simulink model "Plant"  (R2018b)
settings: configuration reference "plant_config" (kept outside this file)
values from neighbouring files (symbols this model uses):
  PLANT_EXPORT = Simulink.Parameter(PLANT_EXPORT_VALUE)    [multicopter_model_init.m]    (also in plant_model_init.m)
undefined symbols (not defined in the file or in its folder): acc_x, acc_x_O, acc_y, acc_y_O, acc_z, acc_z_O, alt, alt_ref, day, DiscIntNeverNeededParam, fixType, flags, gSpeed, gyr_x, gyr_y, gyr_z, h_R, hAcc, headAcc, headMot, height, hMSL, hour, iTOW, lat, lat_ref, lon, lon_ref, M_BO, M_OB, mag_x, mag_y, mag_z, month, nano, Newton, numSV, pDOP, phi, PLANT_CONST, plant_model, pressure, prop_vel, psi, quat, Raphson, reserved1, reserved2, rot_x_B, rot_y_B, rot_z_B, sAcc, sec, Sensor_Model, tAcc, temperature, temprature, theta, timestamp, vAcc ... (+10)
libraries: simulink x6, dspsrcs4 x6, AP_Math x3, Quaternion x3, Rotation x2, aerolibatmos2 x1
(part 1 of 2)
settings Model: Creator=zouji  LastModifiedBy=zouji
settings ConfigSetRef: SourceLocation=Base Workspace

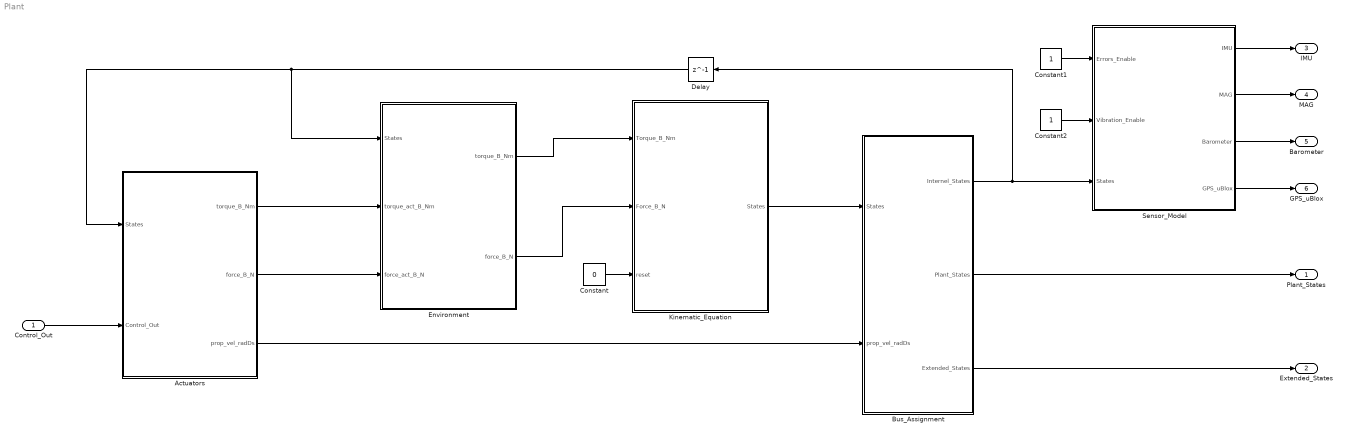
== system Plant ==
  Control_Out : Inport  OutDataTypeStr=Bus: Control_Out_Bus
  Actuators : Subsystem  TreatAsAtomicUnit=on
  Bus_Assignment : Subsystem  TreatAsAtomicUnit=on  mask{lon_0=0.65673, lat_0=-2.1361, hgt_0=4.5}
      mask prompts: lon_0 "init lontitude (rad)"; lat_0 "init latitude (rad)"; hgt_0 "init height (m)"
  Constant : Constant  Value=0  OutDataTypeStr=Inherit: Inherit via back propagation
  Constant1 : Constant  OutDataTypeStr=Inherit: Inherit via back propagation
  Constant2 : Constant  OutDataTypeStr=Inherit: Inherit via back propagation
  Delay : Delay  DelayLength=1
  Environment : Subsystem  TreatAsAtomicUnit=on
  Kinematic_Equation : Subsystem  TreatAsAtomicUnit=on
  Sensor_Model : Subsystem  TreatAsAtomicUnit=on
  Plant_States : Outport  OutDataTypeStr=Bus: Plant_States_Bus
  Extended_States : Outport  Port=2  OutDataTypeStr=Bus: Extended_States_Bus
  IMU : Outport  Port=3  OutDataTypeStr=Bus: IMU_Bus
  MAG : Outport  Port=4  OutDataTypeStr=Bus: MAG_Bus
  Barometer : Outport  Port=5  OutDataTypeStr=Bus: Barometer_Bus
  GPS_uBlox : Outport  Port=6  OutDataTypeStr=Bus: GPS_uBlox_Bus
  wires:
  Kinematic_Equation/1(States) -> Bus_Assignment/1(States)
  Control_Out/1 -> Actuators/2(Control_Out)
  Bus_Assignment/2(Plant_States) -> Plant_States/1
  Constant1/1 -> Sensor_Model/1(Errors_Enable)
  Sensor_Model/1(IMU) -> IMU/1
  Sensor_Model/2(MAG) -> MAG/1
  Sensor_Model/3(Barometer) -> Barometer/1
  Sensor_Model/4(GPS_uBlox) -> GPS_uBlox/1
  Actuators/3(prop_vel_radDs) -> Bus_Assignment/2(prop_vel_radDs)
  Delay/1 -> Environment/1(States), Actuators/1(States)
  Constant2/1 -> Sensor_Model/2(Vibration_Enable)
  Actuators/1(torque_B_Nm) -> Environment/2(torque_act_B_Nm)
  Actuators/2(force_B_N) -> Environment/3(force_act_B_N)
  Environment/1(torque_B_Nm) -> Kinematic_Equation/1(Torque_B_Nm)
  Environment/2(force_B_N) -> Kinematic_Equation/2(Force_B_N)
  Constant/1 -> Kinematic_Equation/3(reset)
  Bus_Assignment/3(Extended_States) -> Extended_States/1
  Bus_Assignment/1(Internel_States) -> Sensor_Model/3(States), Delay/1

== system Plant/Actuators ==
  States : Inport
  Control_Out : Inport  Port=2
  Aerodynamic : Subsystem
  Bus Selector : BusSelector  OutputSignals=Plant_States.rot_x_B,Plant_States.rot_y_B,Plant_States.rot_z_B
  Motors : Subsystem
  Mux : Mux  Inputs=3
  Sum : Sum  Inputs=|++
  torque_B_Nm : Outport
  force_B_N : Outport  Port=2
  prop_vel_radDs : Outport  Port=3
  wires:
  Control_Out/1 -> Motors/1(Control_Out)
  States/1 -> Aerodynamic/1(States), Bus Selector/1
  Motors/1(torque_B_Nm) -> torque_B_Nm/1
  Motors/2(force_B_N) -> Sum/1
  Motors/3(prop_vel_radDs) -> prop_vel_radDs/1
  Bus Selector/1 -> Mux/1  "<rot_x_B>"
  Bus Selector/2 -> Mux/2  "<rot_y_B>"
  Bus Selector/3 -> Mux/3  "<rot_z_B>"
  Mux/1 -> Motors/2(omega_B_radDs)
  Sum/1 -> force_B_N/1
  Aerodynamic/1(aero_force_B_N) -> Sum/2

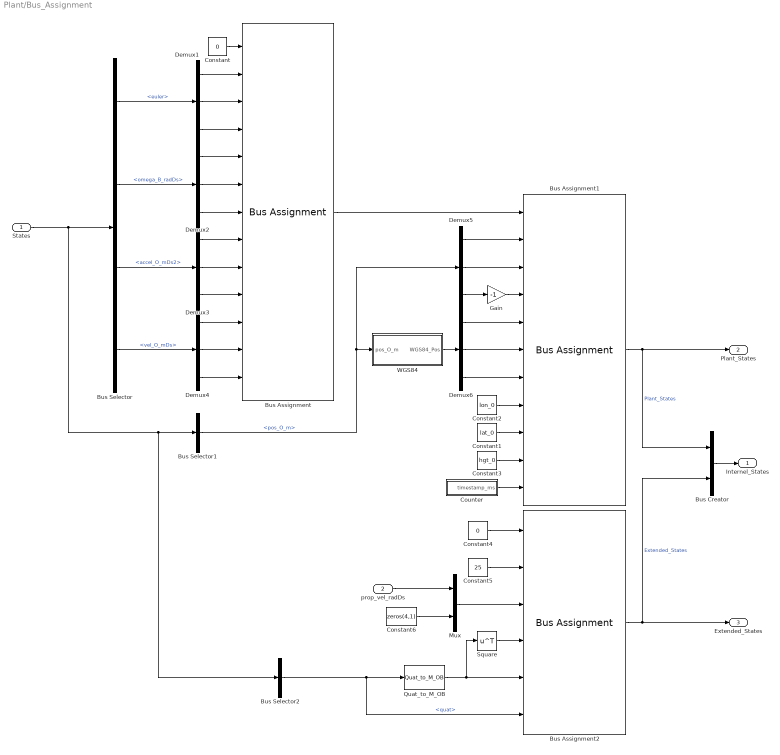
== system Plant/Bus_Assignment ==
  States : Inport
  prop_vel_radDs : Inport  Port=2
  Bus Assignment : BusAssignment  AssignedSignals=phi,theta,psi,rot_x_B,rot_y_B,rot_z_B,acc_x_O,acc_y_O,acc_z_O,vel_x_O,vel_y_O,vel_z_O
  Bus Assignment1 : BusAssignment  AssignedSignals=x_R,y_R,h_R,lat,lon,alt,lon_ref,lat_ref,alt_ref,timestamp
  Bus Assignment2 : BusAssignment  AssignedSignals=temprature,prop_vel,M_BO,M_OB,quat
  Bus Creator : BusCreator  Inputs=2
  Bus Selector : BusSelector  OutputSignals=euler,omega_B_radDs,accel_O_mDs2,vel_O_mDs
  Bus Selector1 : BusSelector  OutputSignals=pos_O_m
  Bus Selector2 : BusSelector  OutputSignals=quat
  Constant : Constant  Value=0  OutDataTypeStr=Bus: Plant_States_Bus
  Constant1 : Constant  Value=lat_0
  Constant2 : Constant  Value=lon_0
  Constant3 : Constant  Value=hgt_0
  Constant4 : Constant  Value=0  OutDataTypeStr=Bus: Extended_States_Bus
  Constant5 : Constant  Value=25  OutDataTypeStr=Inherit: Inherit via back propagation
  Constant6 : Constant  Value=zeros(4,1)  OutDataTypeStr=single
  Counter : Subsystem
  Demux{1..6} (6 alike) : Demux  Outputs=3
  Gain : Gain  Gain=-1  OutDataTypeStr=Inherit: Same as input
  Mux : Mux  Inputs=2
  Quat_to_M_OB : Rotation/Quat_to_M_OB  SystemSampleTime=-1
  Square : Math  Operator=transpose  SaturateOnIntegerOverflow=on
  WGS84 : Subsystem
  Internel_States : Outport
  Plant_States : Outport  Port=2
  Extended_States : Outport  Port=3
  wires:
  Constant/1 -> Bus Assignment/1
  States/1 -> Bus Selector2/1, Bus Selector1/1, Bus Selector/1
  Bus Selector/1 -> Demux1/1  "<euler>"
  Bus Selector/2 -> Demux2/1  "<omega_B_radDs>"
  Bus Selector/3 -> Demux3/1  "<accel_O_mDs2>"
  Bus Selector/4 -> Demux4/1  "<vel_O_mDs>"
  Bus Assignment/1 -> Bus Assignment1/1
  Bus Selector1/1 -> Demux5/1, WGS84/1(pos_O_m)  "<pos_O_m>"
  Bus Assignment1/1 -> Plant_States/1, Bus Creator/1  "Plant_States"
  Quat_to_M_OB/1 -> Bus Assignment2/5, Square/1
  Demux1/2 -> Bus Assignment/3
  prop_vel_radDs/1 -> Mux/1
  Demux5/3 -> Gain/1
  WGS84/1(WGS84_Pos) -> Demux6/1
  Demux1/1 -> Bus Assignment/2
  Demux1/3 -> Bus Assignment/4
  Demux2/1 -> Bus Assignment/5
  Demux2/2 -> Bus Assignment/6
  Demux2/3 -> Bus Assignment/7
  Demux3/1 -> Bus Assignment/8
  Demux3/2 -> Bus Assignment/9
  Demux3/3 -> Bus Assignment/10
  Demux4/1 -> Bus Assignment/11
  Demux4/2 -> Bus Assignment/12
  Demux4/3 -> Bus Assignment/13
  Demux5/2 -> Bus Assignment1/3
  Gain/1 -> Bus Assignment1/4
  Demux5/1 -> Bus Assignment1/2
  Demux6/1 -> Bus Assignment1/5
  Demux6/2 -> Bus Assignment1/6
  Demux6/3 -> Bus Assignment1/7
  Constant2/1 -> Bus Assignment1/8
  Constant1/1 -> Bus Assignment1/9
  Constant3/1 -> Bus Assignment1/10
  Constant4/1 -> Bus Assignment2/1
  Constant5/1 -> Bus Assignment2/2
  Mux/1 -> Bus Assignment2/3
  Constant6/1 -> Mux/2
  Square/1 -> Bus Assignment2/4
  Bus Selector2/1 -> Quat_to_M_OB/1, Bus Assignment2/6  "<quat>"
  Bus Assignment2/1 -> Bus Creator/2, Extended_States/1  "Extended_States"
  Bus Creator/1 -> Internel_States/1
  Counter/1(timestamp_ms) -> Bus Assignment1/11

== system Plant/Environment ==
  States : Inport
  torque_act_B_Nm : Inport  Port=2
  force_act_B_N : Inport  Port=3
  Add : Sum  Inputs=+++
  Add1 : Sum
  Gravity : Subsystem
  Ground_Model : Subsystem
  torque_B_Nm : Outport
  force_B_N : Outport  Port=2
  wires:
  States/1 -> Ground_Model/1(States), Gravity/1(States)
  Gravity/1(g_B_N) -> Add/2
  force_act_B_N/1 -> Add/3
  Ground_Model/2(force_gnd_B_N) -> Add/1
  Add/1 -> force_B_N/1
  Ground_Model/1(torque_gnd_B_Nm) -> Add1/2
  torque_act_B_Nm/1 -> Add1/1
  Add1/1 -> torque_B_Nm/1

== system Plant/Kinematic_Equation ==
  Torque_B_Nm : Inport
  Force_B_N : Inport  Port=2
  reset : Inport  Port=3
  Attitude_Dynamic : Subsystem  mask{Ixx=plant_model.Jxx, Iyy=plant_model.Jyy, Izz=plant_model.Jzz}
  Bus Creator : BusCreator  Inputs=7
  Position_Dynamic : Subsystem  mask{mass=plant_model.mass}
  States : Outport
  wires:
  Attitude_Dynamic/2(omega_B_radDs) -> Bus Creator/2, Position_Dynamic/2(omega_B_radDs)  "omega_B_radDs"
  Attitude_Dynamic/3(quat) -> Bus Creator/3, Position_Dynamic/3(quat)  "quat"
  reset/1 -> Attitude_Dynamic/2(reset), Position_Dynamic/4(vel_reset)
  Bus Creator/1 -> States/1  "states"
  Attitude_Dynamic/1(dot_omega_B_radDs2) -> Bus Creator/1  "dot_omega_B_radDs2"
  Attitude_Dynamic/4(euler) -> Bus Creator/4  "euler"
  Position_Dynamic/1(accel_O_mDs2) -> Bus Creator/5  "accel_O_mDs2"
  Position_Dynamic/2(vel_O_mDs) -> Bus Creator/6  "vel_O_mDs"
  Position_Dynamic/3(pos_NED_O_m) -> Bus Creator/7  "pos_O_m"
  Force_B_N/1 -> Position_Dynamic/1(force_B_N)
  Torque_B_Nm/1 -> Attitude_Dynamic/1(torque_B_Nm)

== system Plant/Sensor_Model ==
  Errors_Enable : Inport  OutDataTypeStr=uint8
  Vibration_Enable : Inport  Port=2  OutDataTypeStr=uint8
  States : Inport  Port=3
  Counter : Subsystem
  Sensor_Barometer : Subsystem  TreatAsAtomicUnit=on
  Sensor_GPS : Subsystem  TreatAsAtomicUnit=on
  Sensor_IMU : Subsystem  TreatAsAtomicUnit=on
  Sensor_MAG : Subsystem  TreatAsAtomicUnit=on
  IMU : Outport
  MAG : Outport  Port=2
  Barometer : Outport  Port=3
  GPS_uBlox : Outport  Port=4
  wires:
  Counter/1(timestamp_ms) -> Sensor_Barometer/3(timestamp_ms), Sensor_MAG/3(timestamp_ms), Sensor_IMU/4(timestamp_ms), Sensor_GPS/3(timestamp_ms)
  States/1 -> Sensor_GPS/1(States), Sensor_Barometer/1(States), Sensor_MAG/1(States), Sensor_IMU/1(States)
  Sensor_Barometer/1(Barometer) -> Barometer/1
  Sensor_MAG/1(Mag) -> MAG/1
  Sensor_IMU/1(IMU) -> IMU/1
  Vibration_Enable/1 -> Sensor_IMU/3(Vibration_Enable)
  Errors_Enable/1 -> Sensor_IMU/2(Errors_Enable), Sensor_GPS/2(Errors_Enable), Sensor_Barometer/2(Errors_Enable), Sensor_MAG/2(Errors_Enable)
  Sensor_GPS/1(GPS_uBlox) -> GPS_uBlox/1

== system Plant/Actuators/Aerodynamic ==
  States : Inport
  Air_Drag : Subsystem
  aero_force_B_N : Outport
  wires:
  States/1 -> Air_Drag/1(Plant_States)
  Air_Drag/1(air_drag_B) -> aero_force_B_N/1

== system Plant/Actuators/Motors ==
  Control_Out : Inport
  omega_B_radDs : Inport  Port=2
  ESCs : Subsystem  mask{T=plant_model.motorT, k=plant_model.motorCr, p=plant_model.motorWb}
  Force : Subsystem
  Torque : Subsystem
  torque_B_Nm : Outport
  force_B_N : Outport  Port=2
  prop_vel_radDs : Outport  Port=3
  wires:
  ESCs/1(rotor_speed_radDs) -> prop_vel_radDs/1, Force/1(rotor_speed_radDs), Torque/1(rotor_speed_radDs)  "prop_vel"
  omega_B_radDs/1 -> Torque/2(omega_B_radDs)
  Control_Out/1 -> ESCs/1(Control_Out)
  Torque/1(torque_B_Nm) -> torque_B_Nm/1
  Force/1(force_B_N) -> force_B_N/1

== system Plant/Bus_Assignment/Counter ==
  note: Careful: If change memory to delay,
      | that model will crash
  Data Type Conversion2 : DataTypeConversion  OutDataTypeStr=uint32
  Memory1 : Memory
  Sum : Sum  Inputs=|++
  dt : Constant  Value=PLANT_EXPORT.period  OutDataTypeStr=uint32
  timestamp_ms : Outport
  wires:
  dt/1 -> Sum/1
  Sum/1 -> Memory1/1
  Memory1/1 -> Sum/2, Data Type Conversion2/1
  Data Type Conversion2/1 -> timestamp_ms/1

== system Plant/Bus_Assignment/WGS84 ==
  pos_O_m : Inport
  Add : Sum
  Data Type Conversion : DataTypeConversion  OutDataTypeStr=double
  Delay : Delay  DelayLength=1
  Delay1 : Delay  DelayLength=1  InitialCondition=[lon_0;lat_0;hgt_0]
  Demux : Demux  Outputs=3
  Divide : Product  Inputs=/*
  Mux : Mux  Inputs=3
  Subtract : Sum  Inputs=+-
  Terminator : Terminator
  WGS84_Derivatives : Subsystem
  Zero_Value_Exclusion : Subsystem  mask{thr=1e-6}
      mask prompts: thr "Threshold"
      mask Display: disp('Exclude Zero');
  WGS84_Pos : Outport
  wires:
  pos_O_m/1 -> Data Type Conversion/1
  Delay/1 -> Subtract/2
  WGS84_Derivatives/1(dx_dlat) -> Mux/1
  Mux/1 -> Zero_Value_Exclusion/1(u)
  Zero_Value_Exclusion/1(y) -> Divide/1
  WGS84_Derivatives/3(dz_dh) -> Mux/3
  WGS84_Derivatives/2(dy_dlon) -> Mux/2
  Subtract/1 -> Divide/2
  Divide/1 -> Add/1
  Delay1/1 -> Demux/1, Add/2
  Add/1 -> Delay1/1, WGS84_Pos/1
  Demux/1 -> WGS84_Derivatives/1(lat_0)
  Demux/3 -> WGS84_Derivatives/2(h_0)
  Demux/2 -> Terminator/1
  Data Type Conversion/1 -> Delay/1, Subtract/1

== system Plant/Environment/Gravity ==
  States : Inport
  Bus Selector4 : BusSelector  OutputSignals=Extended_States.M_BO
  Multiply3 : Product  Multiplication=Matrix(*)
  mg : Constant  Value=[0;0;9.81*plant_model.mass]  OutDataTypeStr=single
  g_B_N : Outport
  wires:
  States/1 -> Bus Selector4/1
  Bus Selector4/1 -> Multiply3/1  "<M_BO>"
  Multiply3/1 -> g_B_N/1
  mg/1 -> Multiply3/2

== system Plant/Environment/Ground_Model ==
  States : Inport
  Bus Selector : BusSelector  OutputSignals=Plant_States.h_R
  Compare To Zero : simulink/Logic and Bit Operations/Compare To Zero  relop=<=  OutDataTypeStr=boolean
  Constant : Constant  Value=[0;0;0]  VectorParams1D=off  OutDataTypeStr=single
  Constant1 : Constant  Value=[0;0;0]  VectorParams1D=off  OutDataTypeStr=single
  Ground_Force : Subsystem
  Ground_Torque : Subsystem
  Switch1 : Switch  Criteria=u2 > Threshold
  Switch2 : Switch  Criteria=u2 > Threshold
  torque_gnd_B_Nm : Outport
  force_gnd_B_N : Outport  Port=2
  wires:
  Compare To Zero/1 -> Switch1/2, Switch2/2
  Constant/1 -> Switch2/3
  Switch2/1 -> force_gnd_B_N/1
  States/1 -> Ground_Force/1(States), Bus Selector/1, Ground_Torque/1(States)
  Bus Selector/1 -> Compare To Zero/1  "<h_R>"
  Ground_Force/1(force_gnd_B_N) -> Switch2/1
  Ground_Torque/1(torque_gnd_B_Nm) -> Switch1/1
  Constant1/1 -> Switch1/3
  Switch1/1 -> torque_gnd_B_Nm/1

== system Plant/Kinematic_Equation/Attitude_Dynamic ==
  torque_B_Nm : Inport
  reset : Inport  Port=2
  Constant1 : Constant  Value=[1;0;0;0]  OutDataTypeStr=single
  Discrete-Time Integrator : DiscreteIntegrator  ExternalReset=level  InitialCondition=[0;0;0]  SampleTime=-1  ICPrevOutput=DiscIntNeverNeededParam  ICPrevScaledInput=DiscIntNeverNeededParam
  Divide : Product  Inputs=/*  Multiplication=Matrix(*)  OutDataTypeStr=Inherit: Same as first input
  Inertia_Matrix : Constant  Value=[Ixx 0 0;0 Iyy 0;0 0 Izz]  OutDataTypeStr=single
  Multiply : Product  Multiplication=Matrix(*)  OutDataTypeStr=Inherit: Same as first input
  Quaternuin_Update : Subsystem
  Sum : Sum  Inputs=|+-  OutDataTypeStr=Inherit: Same as first input
  cross_product : AP_Math/cross_product  SystemSampleTime=-1
  quat to euler : Quaternion/quat to euler  SystemSampleTime=-1
  dot_omega_B_radDs2 : Outport
  omega_B_radDs : Outport  Port=2
  quat : Outport  Port=3
  euler : Outport  Port=4
  wires:
  Constant1/1 -> Quaternuin_Update/3(init_quat)
  quat to euler/1 -> euler/1
  Quaternuin_Update/1(quat) -> quat to euler/1, quat/1
  reset/1 -> Quaternuin_Update/2(reset), Discrete-Time Integrator/2
  Divide/1 -> dot_omega_B_radDs2/1, Discrete-Time Integrator/1  "dot_omega_B_radDs2"
  Sum/1 -> Divide/2
  cross_product/1 -> Sum/2
  torque_B_Nm/1 -> Sum/1
  Multiply/1 -> cross_product/2
  Inertia_Matrix/1 -> Multiply/1, Divide/1
  Discrete-Time Integrator/1 -> omega_B_radDs/1, Multiply/2, cross_product/1, Quaternuin_Update/1(omega_B_radDs)  "omega_B_radDs"

== system Plant/Kinematic_Equation/Position_Dynamic ==
  force_B_N : Inport
  omega_B_radDs : Inport  Port=2
  quat : Inport  Port=3
  vel_reset : Inport  Port=4
  Constant : Constant  Value=0  OutDataTypeStr=Inherit: Inherit via back propagation
  Discrete-Time Integrator : DiscreteIntegrator  ExternalReset=level  InitialCondition=[0;0;0]  SampleTime=-1  ICPrevOutput=DiscIntNeverNeededParam  ICPrevScaledInput=DiscIntNeverNeededParam
  Discrete-Time Integrator1 : DiscreteIntegrator  ExternalReset=level  InitialCondition=[0;0;0]  SampleTime=-1  ICPrevOutput=DiscIntNeverNeededParam  ICPrevScaledInput=DiscIntNeverNeededParam
  Divide : Product  Inputs=*/
  Sum : Sum  Inputs=|+-
  body to earth : Quaternion/body to earth  SystemSampleTime=-1
  cross_product : AP_Math/cross_product  SystemSampleTime=-1
  earth to body : Quaternion/earth to body  SystemSampleTime=-1
  mass : Constant  Value=mass  OutDataTypeStr=single
  accel_O_mDs2 : Outport
  vel_O_mDs : Outport  Port=2
  pos_NED_O_m : Outport  Port=3
  wires:
  force_B_N/1 -> Divide/1
  mass/1 -> Divide/2
  Discrete-Time Integrator/1 -> earth to body/2, vel_O_mDs/1, Discrete-Time Integrator1/1  "vel_O_mDs"
  omega_B_radDs/1 -> cross_product/1
  Divide/1 -> Sum/1
  cross_product/1 -> Sum/2  "centripetal_accel"
  Sum/1 -> body to earth/2
  quat/1 -> earth to body/1, body to earth/1
  Discrete-Time Integrator1/1 -> pos_NED_O_m/1  "pos_O_m"
  body to earth/1 -> accel_O_mDs2/1, Discrete-Time Integrator/1  "accel_O_mDs2"
  vel_reset/1 -> Discrete-Time Integrator/2
  Constant/1 -> Discrete-Time Integrator1/2
  earth to body/1 -> cross_product/2

== system Plant/Sensor_Model/Counter ==
  note: Careful: If change memory to delay,
      | that model will crash
  Data Type Conversion2 : DataTypeConversion  OutDataTypeStr=uint32
  Memory1 : Memory
  Sum : Sum  Inputs=|++
  dt : Constant  Value=PLANT_EXPORT.period  OutDataTypeStr=uint32
  timestamp_ms : Outport
  wires:
  dt/1 -> Sum/1
  Sum/1 -> Memory1/1
  Memory1/1 -> Sum/2, Data Type Conversion2/1
  Data Type Conversion2/1 -> timestamp_ms/1

== system Plant/Sensor_Model/Sensor_Barometer ==
  States : Inport
  Errors_Enable : Inport  Port=2
  timestamp_ms : Inport  Port=3
  Bus_Assignment : Subsystem
  Physical_Model : Subsystem
  Sensor_Model : Subsystem
  Barometer : Outport
  wires:
  Physical_Model/1(Pressure_Pa) -> Sensor_Model/2(u)
  States/1 -> Physical_Model/1(States)
  Sensor_Model/1(y) -> Bus_Assignment/1(Static_Pressure)
  Bus_Assignment/1(Barometer) -> Barometer/1
  Errors_Enable/1 -> Sensor_Model/1(Errors_Enable)
  Physical_Model/2(Temperature_K) -> Bus_Assignment/2(Static_Temperature)
  timestamp_ms/1 -> Bus_Assignment/3(timestamp_ms)

== system Plant/Sensor_Model/Sensor_GPS ==
  States : Inport
  Errors_Enable : Inport  Port=2
  timestamp_ms : Inport  Port=3
  Bus_Assignment : Subsystem
  Physical_Model : Subsystem
  Sensor_Model : Subsystem
  GPS_uBlox : Outport
  wires:
  States/1 -> Physical_Model/1(States)
  Bus_Assignment/1(GPS_uBlox) -> GPS_uBlox/1
  Errors_Enable/1 -> Sensor_Model/1(Errors_Enable)
  Sensor_Model/1(POS_WGS84_meas) -> Bus_Assignment/1(POS_WGS84)
  Sensor_Model/2(VEL_O_meas) -> Bus_Assignment/2(VEL_O_meas)
  Sensor_Model/3(numSV) -> Bus_Assignment/3(numSV)
  Sensor_Model/4(fixType) -> Bus_Assignment/4(fixType)
  Sensor_Model/5(h_Acc_m) -> Bus_Assignment/5(h_Acc_m)
  Physical_Model/1(POS_O_WGS84) -> Sensor_Model/2(POS_WGS84)
  Physical_Model/2(VEL_O_mDs) -> Sensor_Model/3(VEL_O)
  Sensor_Model/6(v_Acc_m) -> Bus_Assignment/6(v_Acc_m)
  Sensor_Model/7(s_Acc_mDs) -> Bus_Assignment/7(s_Acc_m)
  timestamp_ms/1 -> Bus_Assignment/8(timestamp_ms)

== system Plant/Sensor_Model/Sensor_IMU ==
  States : Inport
  Errors_Enable : Inport  Port=2
  Vibration_Enable : Inport  Port=3
  timestamp_ms : Inport  Port=4
  Accelerometer : Subsystem
  Bus_Assignment : Subsystem
  Gyroscope : Subsystem
  IMU : Outport
  wires:
  Gyroscope/1(Gyro_Raw) -> Bus_Assignment/1(Gyro_Raw)
  Bus_Assignment/1(IMU) -> IMU/1
  Vibration_Enable/1 -> Accelerometer/3(Vibration_Enbale), Gyroscope/3(Vibration_Enable)
  States/1 -> Accelerometer/1(States), Gyroscope/1(States)
  Errors_Enable/1 -> Accelerometer/2(Errors_Enables), Gyroscope/2(Errors_Enable)
  Accelerometer/1(Acc_Raw) -> Bus_Assignment/2(Acc_Raw)
  timestamp_ms/1 -> Bus_Assignment/3(timestamp_ms)

== system Plant/Sensor_Model/Sensor_MAG ==
  States : Inport
  Errors_Enable : Inport  Port=2
  timestamp_ms : Inport  Port=3
  Bus_Assignment : Subsystem
  Sensor_Magnetometer : Subsystem
  Mag : Outport
  wires:
  Sensor_Magnetometer/1(Mag_Raw) -> Bus_Assignment/1(Mag_Raw)
  Bus_Assignment/1(MAG) -> Mag/1
  States/1 -> Sensor_Magnetometer/1(States)
  Errors_Enable/1 -> Sensor_Magnetometer/2(Errors_Enable)
  timestamp_ms/1 -> Bus_Assignment/2(timestamp_ms)

== system Plant/Actuators/Aerodynamic/Air_Drag ==
  Plant_States : Inport
  Bus Selector : BusSelector  OutputSignals=Plant_States.psi,Plant_States.vel_x_O,Plant_States.vel_y_O,Plant_States.vel_z_O
  Bus Selector1 : BusSelector  OutputSignals=Extended_States.M_BO
  Gain : Gain  Gain=-0.15
  M_CO : Rotation/M_CO  SystemSampleTime=-1
  Multiply : Product  Multiplication=Matrix(*)
  Multiply1 : Product  Multiplication=Matrix(*)
  Multiply2 : Product  Multiplication=Matrix(*)
  Mux : Mux  Inputs=3
  Square : Math  Operator=transpose  SaturateOnIntegerOverflow=on
  air_drag_B : Outport
  wires:
  Bus Selector/2 -> Mux/1  "<vel_x_O>"
  Bus Selector/3 -> Mux/2  "<vel_y_O>"
  Gain/1 -> Multiply1/2
  Mux/1 -> Multiply/2
  Plant_States/1 -> Bus Selector1/1, Bus Selector/1
  Bus Selector/4 -> Mux/3  "<vel_z_O>"
  Multiply/1 -> Gain/1
  Bus Selector/1 -> M_CO/1  "<psi>"
  M_CO/1 -> Square/1, Multiply/1
  Square/1 -> Multiply1/1
  Multiply1/1 -> Multiply2/2
  Bus Selector1/1 -> Multiply2/1  "<M_BO>"
  Multiply2/1 -> air_drag_B/1

== system Plant/Actuators/Motors/ESCs ==
  Control_Out : Inport
  Bus Selector : BusSelector  OutputSignals=actuator_cmd
  Calculate_Rotor_Speed : Subsystem
  Discrete Filter : DiscreteFilter  Denominator=[1 T]
  Selector : Selector  InputPortWidth=16  IndexOptions=Index vector (dialog)  Indices=[1:4]  OutputSizes=1
  Signal_Unified : Subsystem
  rotor_speed_radDs : Outport
  wires:
  Discrete Filter/1 -> rotor_speed_radDs/1
  Control_Out/1 -> Bus Selector/1
  Selector/1 -> Signal_Unified/1(Control_Out)
  Signal_Unified/1(u0) -> Calculate_Rotor_Speed/1(u0)
  Calculate_Rotor_Speed/1(omega_B_radPs) -> Discrete Filter/1
  Bus Selector/1 -> Selector/1  "<actuator_cmd>"

== system Plant/Actuators/Motors/Force ==
  rotor_speed_radDs : Inport
  Constant : Constant  Value=0  OutDataTypeStr=single
  Constant1 : Constant  Value=0  OutDataTypeStr=single
  Gain : Gain  Gain=-1  OutDataTypeStr=Inherit: Same as input
  Mux : Mux  Inputs=3
  Sum of Elements : Sum  Inputs=+
  Thrust : Subsystem  mask{cT=plant_model.Ct}
  force_B_N : Outport
  wires:
  rotor_speed_radDs/1 -> Thrust/1(rotor_speed_radDs)
  Sum of Elements/1 -> Gain/1
  Thrust/1(thrust_B_N) -> Sum of Elements/1
  Gain/1 -> Mux/3
  Mux/1 -> force_B_N/1
  Constant/1 -> Mux/1
  Constant1/1 -> Mux/2

== system Plant/Actuators/Motors/Torque ==
  rotor_speed_radDs : Inport
  omega_B_radDs : Inport  Port=2
  Gyroscopic_Torque : Subsystem  mask{Im=plant_model.motorJm}
  Rotor_Generated_Torque : Subsystem  mask{L=plant_model.R*sin(pi/4), cT=plant_model.Ct, cQ=plant_model.Cm}
  Sum : Sum  Inputs=|++
  torque_B_Nm : Outport
  wires:
  rotor_speed_radDs/1 -> Gyroscopic_Torque/1(rotor_speed_radDs), Rotor_Generated_Torque/1(rotor_speed_radDs)
  omega_B_radDs/1 -> Gyroscopic_Torque/2(omega_B_radDs)
  Rotor_Generated_Torque/1(rotor_torque) -> Sum/1
  Sum/1 -> torque_B_Nm/1
  Gyroscopic_Torque/1(gyroscopic_torque) -> Sum/2

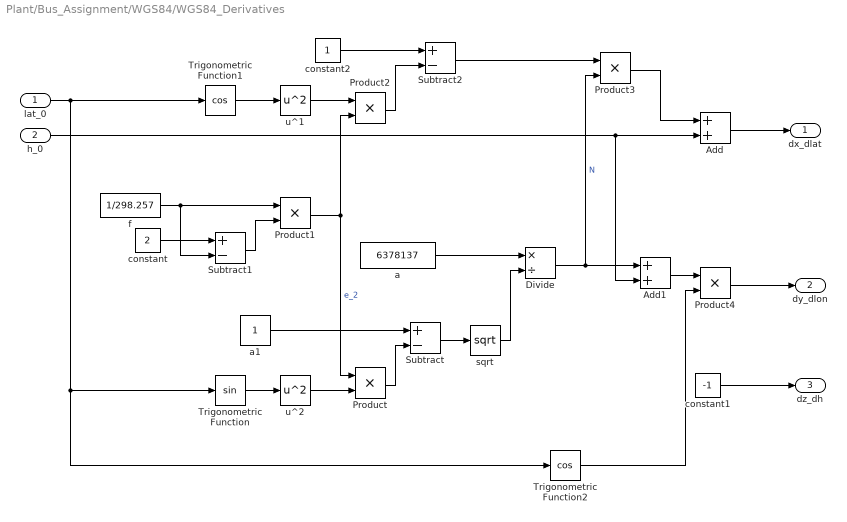
== system Plant/Bus_Assignment/WGS84/WGS84_Derivatives ==
  lat_0 : Inport
  h_0 : Inport  Port=2
  Add : Sum
  Add1 : Sum
  Divide : Product  Inputs=*/
  Product{,1..4} (5 alike) : Product  RndMeth=Zero
  Subtract : Sum  Inputs=+-
  Subtract1 : Sum  Inputs=+-
  Subtract2 : Sum  Inputs=+-
  Trigonometric Function : Trigonometry
  Trigonometric Function1 : Trigonometry  Operator=cos
  Trigonometric Function2 : Trigonometry  Operator=cos
  a : Constant  Value=6378137
  a1 : Constant
  constant : Constant  Value=2
  constant1 : Constant  Value=-1
  constant2 : Constant
  f : Constant  Value=1/298.257
  sqrt : Math  Operator=sqrt  SaturateOnIntegerOverflow=on
  u^1 : Math  Operator=square  SaturateOnIntegerOverflow=on
  u^2 : Math  Operator=square  SaturateOnIntegerOverflow=on
  dx_dlat : Outport
  dy_dlon : Outport  Port=2
  dz_dh : Outport  Port=3  InitialOutput=1
  wires:
  constant1/1 -> dz_dh/1
  Product4/1 -> dy_dlon/1
  Add1/1 -> Product4/1
  Trigonometric Function2/1 -> Product4/2
  Product3/1 -> Add/1
  Subtract2/1 -> Product3/1
  Product2/1 -> Subtract2/2
  u^1/1 -> Product2/1
  Trigonometric Function1/1 -> u^1/1
  constant2/1 -> Subtract2/1
  h_0/1 -> Add1/2, Add/2
  Add/1 -> dx_dlat/1
  Divide/1 -> Add1/1, Product3/2  "N"
  sqrt/1 -> Divide/2
  Product1/1 -> Product2/2, Product/1  "e_2"
  Subtract1/1 -> Product1/2
  constant/1 -> Subtract1/1
  f/1 -> Subtract1/2, Product1/1
  Product/1 -> Subtract/2
  Subtract/1 -> sqrt/1
  a1/1 -> Subtract/1
  u^2/1 -> Product/2
  Trigonometric Function/1 -> u^2/1
  lat_0/1 -> Trigonometric Function2/1, Trigonometric Function/1, Trigonometric Function1/1
  a/1 -> Divide/1

== system Plant/Bus_Assignment/WGS84/Zero_Value_Exclusion ==
  u : Inport
  Abs : Abs
  Constant : Constant
  Product : Product  RndMeth=Zero
  Saturation : Saturate  UpperLimit=10e7  LowerLimit=thr
  Sign : Signum
  Switch : Switch  Criteria=u2 ~= 0
  y : Outport
  wires:
  u/1 -> Sign/1, Abs/1
  Abs/1 -> Saturation/1
  Saturation/1 -> Product/1
  Sign/1 -> Switch/2, Switch/1
  Product/1 -> y/1
  Switch/1 -> Product/2
  Constant/1 -> Switch/3

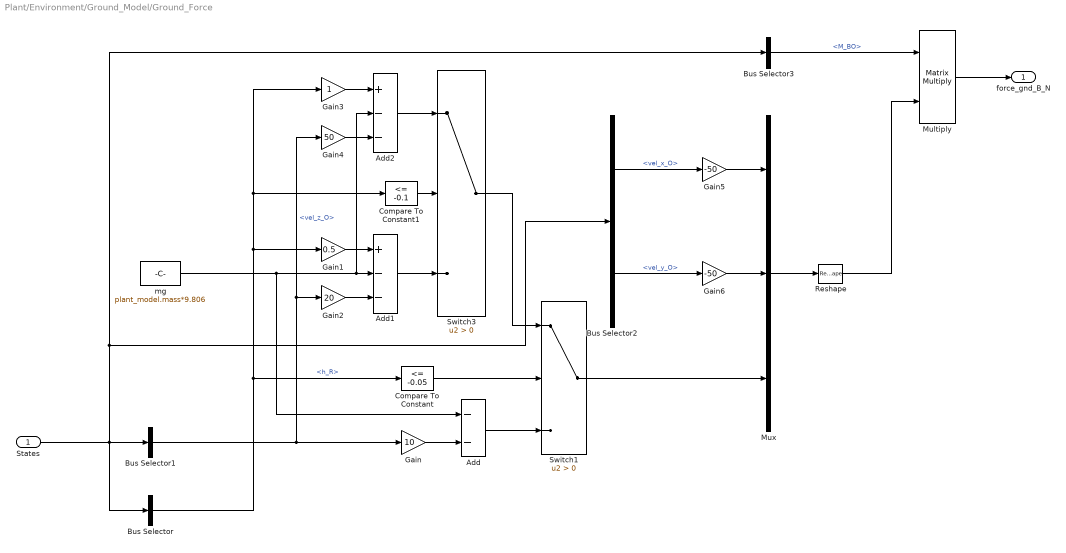
== system Plant/Environment/Ground_Model/Ground_Force ==
  States : Inport
  Add : Sum  Inputs=--
  Add1 : Sum  Inputs=+--
  Add2 : Sum  Inputs=+--
  Bus Selector : BusSelector  OutputSignals=Plant_States.h_R
  Bus Selector1 : BusSelector  OutputSignals=Plant_States.vel_z_O
  Bus Selector2 : BusSelector  OutputSignals=Plant_States.vel_x_O,Plant_States.vel_y_O
  Bus Selector3 : BusSelector  OutputSignals=Extended_States.M_BO
  Compare To Constant : simulink/Logic and Bit Operations/Compare To Constant  relop=<=  const=-0.05  OutDataTypeStr=boolean
  Compare To Constant1 : simulink/Logic and Bit Operations/Compare To Constant  relop=<=  const=-0.1  OutDataTypeStr=boolean
  Gain : Gain  Gain=10
  Gain1 : Gain  Gain=0.5
  Gain2 : Gain  Gain=20
  Gain3 : Gain
  Gain4 : Gain  Gain=50
  Gain5 : Gain  Gain=-50
  Gain6 : Gain  Gain=-50
  Multiply : Product  Multiplication=Matrix(*)
  Mux : Mux  Inputs=3
  Reshape : Reshape  OutputDimensionality=Customize  OutputDimensions=[3,1]
  Switch1 : Switch  Criteria=u2 > Threshold
  Switch3 : Switch  Criteria=u2 > Threshold
  mg : Constant  Value=plant_model.mass*9.806  OutDataTypeStr=single
  force_gnd_B_N : Outport
  wires:
  Switch1/1 -> Mux/3
  Bus Selector/1 -> Compare To Constant/1, Gain1/1, Gain3/1, Compare To Constant1/1  "<h_R>"
  Bus Selector1/1 -> Gain4/1, Gain2/1, Gain/1  "<vel_z_O>"
  Switch3/1 -> Switch1/1
  Gain1/1 -> Add1/1
  Gain5/1 -> Mux/1
  Gain3/1 -> Add2/1
  Compare To Constant/1 -> Switch1/2
  mg/1 -> Add/1, Add2/2, Add1/2
  Gain/1 -> Add/2
  Bus Selector2/2 -> Gain6/1  "<vel_y_O>"
  Gain2/1 -> Add1/3
  Add/1 -> Switch1/3
  Add2/1 -> Switch3/1
  Bus Selector2/1 -> Gain5/1  "<vel_x_O>"
  Gain6/1 -> Mux/2
  Compare To Constant1/1 -> Switch3/2
  Gain4/1 -> Add2/3
  Add1/1 -> Switch3/3
  Bus Selector3/1 -> Multiply/1  "<M_BO>"
  Mux/1 -> Reshape/1
  Multiply/1 -> force_gnd_B_N/1
  Reshape/1 -> Multiply/2
  States/1 -> Bus Selector/1, Bus Selector1/1, Bus Selector3/1, Bus Selector2/1

== system Plant/Environment/Ground_Model/Ground_Torque ==
  States : Inport
  Bus Selector1 : BusSelector  OutputSignals=Extended_States.quat
  Bus Selector2 : BusSelector  OutputSignals=Plant_States.rot_x_B,Plant_States.rot_y_B,Plant_States.rot_z_B
  Constant : Constant  Value=0  OutDataTypeStr=single
  Gain : Gain  Gain=200
  Gain1 : Gain  Gain=10
  Mux : Mux  Inputs=2
  Mux1 : Mux  Inputs=3
  Reshape1 : Reshape  OutputDimensionality=Customize  OutputDimensions=[3,1]
  Selector : Selector  InputPortWidth=4  IndexOptions=Index vector (dialog)  Indices=[2:3]  OutputSizes=1
  Subtract : Sum  Inputs=--
  torque_gnd_B_Nm : Outport
  wires:
  Reshape1/1 -> torque_gnd_B_Nm/1
  States/1 -> Bus Selector2/1, Bus Selector1/1
  Bus Selector1/1 -> Selector/1  "<quat>"
  Selector/1 -> Mux/1
  Gain/1 -> Subtract/1
  Subtract/1 -> Reshape1/1
  Bus Selector2/1 -> Mux1/1  "<rot_x_B>"
  Bus Selector2/2 -> Mux1/2  "<rot_y_B>"
  Bus Selector2/3 -> Mux1/3  "<rot_z_B>"
  Mux1/1 -> Gain1/1
  Gain1/1 -> Subtract/2
  Constant/1 -> Mux/2
  Mux/1 -> Gain/1

== system Plant/Kinematic_Equation/Attitude_Dynamic/Quaternuin_Update ==
  omega_B_radDs : Inport
  reset : Inport  Port=2
  init_quat : Inport  Port=3
  Discrete-Time Integrator : DiscreteIntegrator  ExternalReset=level  InitialConditionSource=external  SampleTime=-1  ICPrevOutput=DiscIntNeverNeededParam  ICPrevScaledInput=DiscIntNeverNeededParam
  Gain : Gain  Gain=0.5  OutDataTypeStr=Inherit: Same as input
  Multiply : Product  Multiplication=Matrix(*)  OutDataTypeStr=Inherit: Same as first input
  Quaternion_Update_Maxtrix : Subsystem
  quat : Outport
  wires:
  Gain/1 -> Discrete-Time Integrator/1  "dot_q"
  Discrete-Time Integrator/1 -> quat/1, Multiply/2
  init_quat/1 -> Discrete-Time Integrator/3
  reset/1 -> Discrete-Time Integrator/2
  Multiply/1 -> Gain/1
  Quaternion_Update_Maxtrix/1(W) -> Multiply/1
  omega_B_radDs/1 -> Quaternion_Update_Maxtrix/1(omega_B_radDs)

== system Plant/Sensor_Model/Sensor_Barometer/Bus_Assignment ==
  Static_Pressure : Inport  Unit=N/m^2
  Static_Temperature : Inport  Port=2  Unit=K
  timestamp_ms : Inport  Port=3
  Bus Assignment : BusAssignment  AssignedSignals=timestamp,pressure,temperature
  Constant : Constant  Value=0  OutDataTypeStr=Bus: Barometer_Bus
  Constant2 : Constant  Value=273.15
  Data Type Conversion : DataTypeConversion  OutDataTypeStr=single
  Data Type Conversion1 : DataTypeConversion  OutDataTypeStr=single
  Rate Transition : RateTransition  OutPortSampleTime=0.01
  Sum1 : Sum  Inputs=|+-
  Barometer : Outport
  wires:
  Data Type Conversion1/1 -> Bus Assignment/4
  Constant/1 -> Bus Assignment/1
  Data Type Conversion/1 -> Bus Assignment/3
  Bus Assignment/1 -> Rate Transition/1
  Static_Pressure/1 -> Data Type Conversion/1
  Static_Temperature/1 -> Sum1/1
  Rate Transition/1 -> Barometer/1
  Sum1/1 -> Data Type Conversion1/1
  Constant2/1 -> Sum1/2
  timestamp_ms/1 -> Bus Assignment/2

== system Plant/Sensor_Model/Sensor_Barometer/Physical_Model ==
  States : Inport
  Bus Selector1 : BusSelector  OutputSignals=Plant_States.alt
  Data Type Conversion : DataTypeConversion  OutDataTypeStr=single
  ISA Atmosphere Model : aerolibatmos2/ISA Atmosphere Model  custom=off  g=9.80665  gamma=1.4  R=287.0531  L=0.0065  h_trop=11000  h_strat=20000  rho0=1.225  P0=101325  T0=288.15  h0=0
      settings: SourceProductName=Aerospace Blockset
  Terminator : Terminator
  Terminator1 : Terminator
  Pressure_Pa : Outport
  Temperature_K : Outport  Port=2
  wires:
  States/1 -> Bus Selector1/1
  ISA Atmosphere Model/1 -> Temperature_K/1
  ISA Atmosphere Model/2 -> Terminator1/1
  ISA Atmosphere Model/4 -> Terminator/1
  Bus Selector1/1 -> Data Type Conversion/1  "<alt>"
  ISA Atmosphere Model/3 -> Pressure_Pa/1
  Data Type Conversion/1 -> ISA Atmosphere Model/1

== system Plant/Sensor_Model/Sensor_Barometer/Sensor_Model ==
  Errors_Enable : Inport
  u : Inport  Port=2
  Add : Sum  InputSameDT=on  OutDataTypeStr=Inherit: Same as first input
  Random Source : dspsrcs4/Random Source  SrcType=Gaussian  NormMethod=Ziggurat  CltLength=12  MinVal=0  MaxVal=1  MeanVal=0  VarVal=Sensor_Model.Baro.Variance  RepMode=Repeatable  rawSeed=1  IsInherit=off  SampMode=Discrete  SampTime=-1  SampFrame=1  DataType=Single  OutComplex=Real  OutputFrames=off
  Routing : Subsystem
  Saturation : Saturate  UpperLimit=Sensor_Model.Baro.Upper_limit  LowerLimit=Sensor_Model.Baro.Lower_limit  OutDataTypeStr=single
  Sensor_Error : Subsystem
  y : Outport
  wires:
  u/1 -> Routing/2(output_clean), Sensor_Error/1(u)
  Routing/1(y) -> y/1
  Errors_Enable/1 -> Routing/1(Errors_Enable)
  Add/1 -> Routing/3(output_error)
  Saturation/1 -> Add/1
  Sensor_Error/1(y) -> Saturation/1
  Random Source/1 -> Add/2

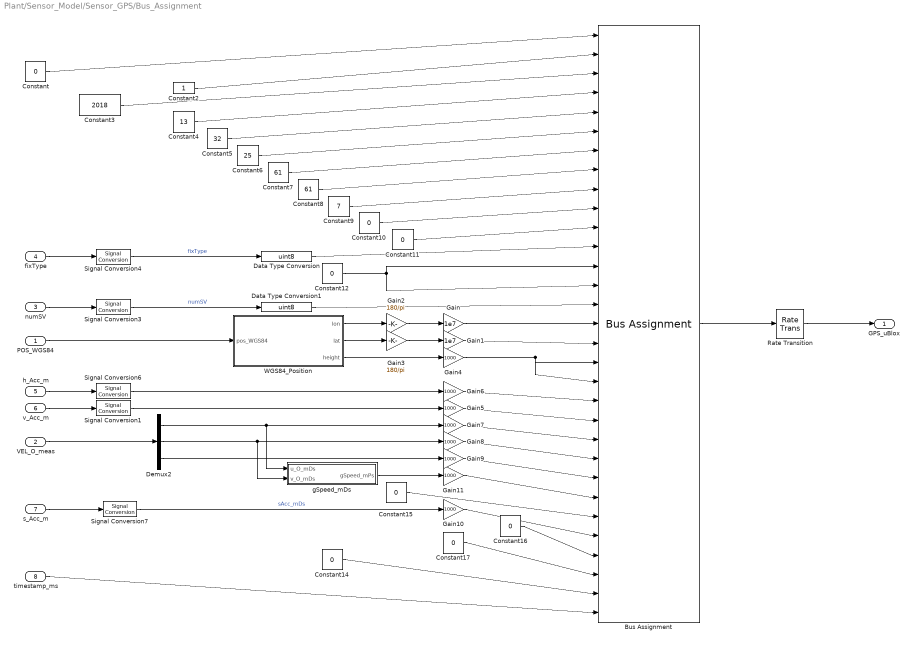
== system Plant/Sensor_Model/Sensor_GPS/Bus_Assignment ==
  POS_WGS84 : Inport
  VEL_O_meas : Inport  Port=2  Unit=m/s
  numSV : Inport  Port=3
  fixType : Inport  Port=4
  h_Acc_m : Inport  Port=5
  v_Acc_m : Inport  Port=6
  s_Acc_m : Inport  Port=7
  timestamp_ms : Inport  Port=8
  Bus Assignment : BusAssignment  AssignedSignals=iTOW,year,month,day,hour,min,sec,valid,tAcc,nano,fixType,flags,reserved1,numSV,lon,lat,height,hMSL,hAcc,vAcc,velN,velE,velD,gSpeed,headMot,sAcc,headAcc,pDOP,reserved2,timestamp
  Constant : Constant  Value=0  OutDataTypeStr=Bus: GPS_uBlox_Bus
  Constant10 : Constant  Value=0  OutDataTypeStr=uint32
  Constant11 : Constant  Value=0  OutDataTypeStr=int32
  Constant12 : Constant  Value=0  OutDataTypeStr=uint8
  Constant14 : Constant  Value=0  OutDataTypeStr=uint16
  Constant15 : Constant  Value=0  OutDataTypeStr=int32
  Constant16 : Constant  Value=0  OutDataTypeStr=uint32
  Constant17 : Constant  Value=0  OutDataTypeStr=uint16
  Constant2 : Constant  OutDataTypeStr=uint32
  Constant3 : Constant  Value=2018  OutDataTypeStr=uint16
  Constant4 : Constant  Value=13  OutDataTypeStr=uint8
  Constant5 : Constant  Value=32  OutDataTypeStr=uint8
  Constant6 : Constant  Value=25  OutDataTypeStr=uint8
  Constant7 : Constant  Value=61  OutDataTypeStr=uint8
  Constant8 : Constant  Value=61  OutDataTypeStr=uint8
  Constant9 : Constant  Value=7  OutDataTypeStr=uint8
  Data Type Conversion : DataTypeConversion  OutDataTypeStr=uint8
  Data Type Conversion1 : DataTypeConversion  OutDataTypeStr=uint8
  Demux2 : Demux  Outputs=3
  Gain : Gain  Gain=1e7  OutDataTypeStr=int32
      settings: AttributesFormatString=Gain: %<Gain>
  Gain1 : Gain  Gain=1e7  OutDataTypeStr=int32
      settings: AttributesFormatString=Gain: %<Gain>
  Gain10 : Gain  Gain=1000  OutDataTypeStr=uint32
      settings: AttributesFormatString=Gain: %<Gain>
  Gain{4,7..9,11} (5 alike) : Gain  Gain=1000  OutDataTypeStr=int32
      settings: AttributesFormatString=Gain: %<Gain>
  Gain2 : Gain  Gain=180/pi
      settings: AttributesFormatString=Gain: %<Gain>
  Gain3 : Gain  Gain=180/pi
      settings: AttributesFormatString=Gain: %<Gain>
  Gain5 : Gain  Gain=1000  OutDataTypeStr=uint32
      settings: AttributesFormatString=Gain: %<Gain>
  Gain6 : Gain  Gain=1000  OutDataTypeStr=uint32
      settings: AttributesFormatString=Gain: %<Gain>
  Rate Transition : RateTransition  OutPortSampleTime=0.1
  Signal Conversion{1,3..4,6..7} (5 alike) : SignalConversion  OverrideOpt=off
  WGS84_Position : Subsystem
  gSpeed_mDs : Subsystem
  GPS_uBlox : Outport
  wires:
  s_Acc_m/1 -> Signal Conversion7/1
  h_Acc_m/1 -> Signal Conversion6/1
  fixType/1 -> Signal Conversion4/1
  numSV/1 -> Signal Conversion3/1
  VEL_O_meas/1 -> Demux2/1
  Gain5/1 -> Bus Assignment/21
  Constant15/1 -> Bus Assignment/26
  Data Type Conversion/1 -> Bus Assignment/12
  Constant17/1 -> Bus Assignment/29
  Gain4/1 -> Bus Assignment/19, Bus Assignment/18
  Constant16/1 -> Bus Assignment/28
  Gain3/1 -> Gain1/1
  Signal Conversion6/1 -> Gain6/1
  Gain6/1 -> Bus Assignment/20
  Gain11/1 -> Bus Assignment/25
  Gain8/1 -> Bus Assignment/23
  Gain7/1 -> Bus Assignment/22
  Gain10/1 -> Bus Assignment/27
  Constant/1 -> Bus Assignment/1
  Constant8/1 -> Bus Assignment/8
  Gain2/1 -> Gain/1
  Constant4/1 -> Bus Assignment/4
  Constant11/1 -> Bus Assignment/11
  Constant10/1 -> Bus Assignment/10
  Constant9/1 -> Bus Assignment/9
  Constant3/1 -> Bus Assignment/3
  Constant6/1 -> Bus Assignment/6
  Bus Assignment/1 -> Rate Transition/1
  Gain9/1 -> Bus Assignment/24
  Constant12/1 -> Bus Assignment/14, Bus Assignment/13
  Constant14/1 -> Bus Assignment/30
  gSpeed_mDs/1(gSpeed_mPs) -> Gain11/1
  Constant5/1 -> Bus Assignment/5
  Gain/1 -> Bus Assignment/16
  Data Type Conversion1/1 -> Bus Assignment/15
  Constant2/1 -> Bus Assignment/2
  Gain1/1 -> Bus Assignment/17
  Constant7/1 -> Bus Assignment/7
  Signal Conversion7/1 -> Gain10/1  "sAcc_mDs"
  Demux2/1 -> gSpeed_mDs/1(u_O_mDs), Gain7/1
  Demux2/2 -> Gain8/1, gSpeed_mDs/2(v_O_mDs)
  Demux2/3 -> Gain9/1
  POS_WGS84/1 -> WGS84_Position/1(pos_WGS84)
  WGS84_Position/1(lon) -> Gain2/1
  WGS84_Position/2(lat) -> Gain3/1
  WGS84_Position/3(height) -> Gain4/1
  Signal Conversion3/1 -> Data Type Conversion1/1  "numSV"
  Signal Conversion4/1 -> Data Type Conversion/1  "fixType"
  v_Acc_m/1 -> Signal Conversion1/1
  Signal Conversion1/1 -> Gain5/1
  Rate Transition/1 -> GPS_uBlox/1
  timestamp_ms/1 -> Bus Assignment/31

== system Plant/Sensor_Model/Sensor_GPS/Physical_Model ==
  note: Transfer Delay
  States : Inport
  Bus Selector : BusSelector  OutputSignals=Plant_States.lon,Plant_States.lat,Plant_States.alt
  Bus Selector1 : BusSelector  OutputSignals=Plant_States.vel_x_O,Plant_States.vel_y_O,Plant_States.vel_z_O
  Delay : Delay  DelayLength=150/(PLANT_CONST.dt*1e3)
  Delay1 : Delay  DelayLength=100/(PLANT_CONST.dt*1e3)
  Vector Concatenate : Concatenate  NumInputs=3  Mode=Multidimensional array
  Vector Concatenate1 : Concatenate  NumInputs=3  Mode=Multidimensional array
  POS_O_WGS84 : Outport  Unit=rad/s
  VEL_O_mDs : Outport  Port=2  Unit=m/s  PortDimensions=[3 1]
  wires:
  Bus Selector/3 -> Vector Concatenate/3  "<alt>"
  Bus Selector/2 -> Vector Concatenate/2  "<lat>"
  Bus Selector/1 -> Vector Concatenate/1  "<lon>"
  Vector Concatenate/1 -> Delay/1
  Bus Selector1/2 -> Vector Concatenate1/2  "<vel_y_O>"
  Bus Selector1/3 -> Vector Concatenate1/3  "<vel_z_O>"
  States/1 -> Bus Selector1/1, Bus Selector/1
  Vector Concatenate1/1 -> Delay1/1
  Bus Selector1/1 -> Vector Concatenate1/1  "<vel_x_O>"
  Delay/1 -> POS_O_WGS84/1
  Delay1/1 -> VEL_O_mDs/1

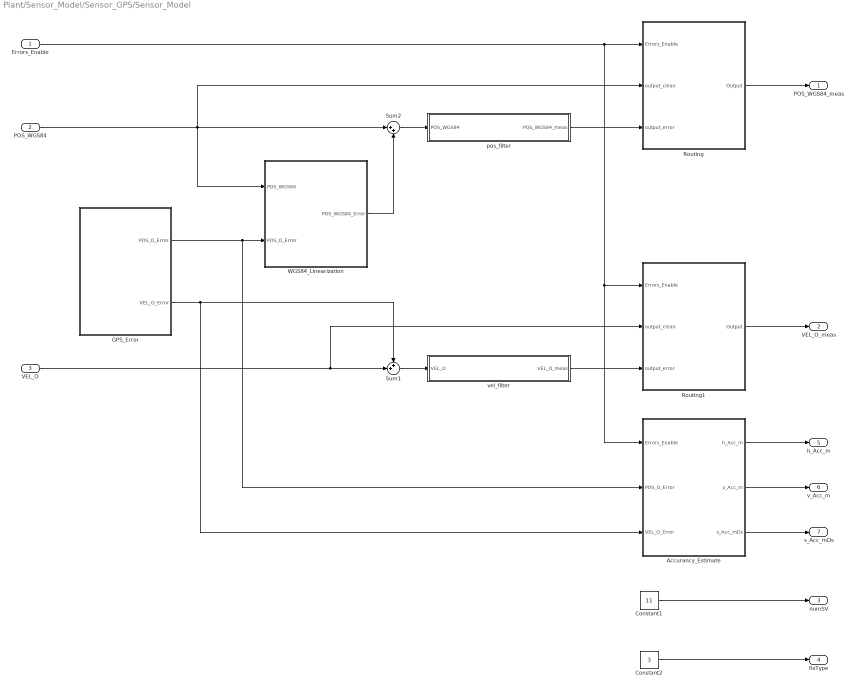
== system Plant/Sensor_Model/Sensor_GPS/Sensor_Model ==
  Errors_Enable : Inport
  POS_WGS84 : Inport  Port=2
  VEL_O : Inport  Port=3
  Accurancy_Estimate : Subsystem
  Constant1 : Constant  Value=11  OutDataTypeStr=Inherit: Inherit via back propagation
  Constant2 : Constant  Value=3  OutDataTypeStr=Inherit: Inherit via back propagation
  GPS_Error : Subsystem
  Routing : Subsystem
  Routing1 : Subsystem
  Sum1 : Sum  Inputs=++|
  Sum2 : Sum  Inputs=|++
  WGS84_Linearization : Subsystem
  pos_filter : Subsystem
  vel_filter : Subsystem
  POS_WGS84_meas : Outport
  VEL_O_meas : Outport  Port=2
  numSV : Outport  Port=3
  fixType : Outport  Port=4
  h_Acc_m : Outport  Port=5
  v_Acc_m : Outport  Port=6
  s_Acc_mDs : Outport  Port=7
  wires:
  Constant2/1 -> fixType/1
  Constant1/1 -> numSV/1
  Routing/1(Output) -> POS_WGS84_meas/1
  POS_WGS84/1 -> Routing/2(output_clean), WGS84_Linearization/1(POS_WGS84), Sum2/1
  Routing1/1(Output) -> VEL_O_meas/1
  VEL_O/1 -> Routing1/2(output_clean), Sum1/2
  Errors_Enable/1 -> Accurancy_Estimate/1(Errors_Enable), Routing1/1(Errors_Enable), Routing/1(Errors_Enable)
  vel_filter/1(VEL_O_meas) -> Routing1/3(output_error)
  pos_filter/1(POS_WGS84_meas) -> Routing/3(output_error)
  Sum2/1 -> pos_filter/1(POS_WGS84)
  GPS_Error/1(POS_O_Error) -> Accurancy_Estimate/2(POS_O_Error), WGS84_Linearization/2(POS_O_Error)
  Sum1/1 -> vel_filter/1(VEL_O)
  GPS_Error/2(VEL_O_Error) -> Accurancy_Estimate/3(VEL_O_Error), Sum1/1
  WGS84_Linearization/1(POS_WGS84_Error) -> Sum2/2
  Accurancy_Estimate/1(h_Acc_m) -> h_Acc_m/1
  Accurancy_Estimate/3(s_Acc_mDs) -> s_Acc_mDs/1
  Accurancy_Estimate/2(v_Acc_m) -> v_Acc_m/1

== system Plant/Sensor_Model/Sensor_IMU/Accelerometer ==
  States : Inport
  Errors_Enables : Inport  Port=2
  Vibration_Enbale : Inport  Port=3
  Bus Assignment : Subsystem
  Physical_Model : Subsystem
  Sensor_Model : Subsystem
  Acc_Raw : Outport
  wires:
  Sensor_Model/1(y) -> Bus Assignment/1(Output)
  States/1 -> Physical_Model/1(States)
  Physical_Model/1(sfor_B_mPs2) -> Sensor_Model/2(u)
  Bus Assignment/1(Acc_Raw) -> Acc_Raw/1
  Errors_Enables/1 -> Sensor_Model/1(Errors_Enables)
  Vibration_Enbale/1 -> Physical_Model/2(Vibration_Enbale)

== system Plant/Sensor_Model/Sensor_IMU/Bus_Assignment ==
  Gyro_Raw : Inport
  Acc_Raw : Inport  Port=2
  timestamp_ms : Inport  Port=3
  Bus Assignment : BusAssignment  AssignedSignals=timestamp,gyr_x,gyr_y,gyr_z,acc_x,acc_y,acc_z
  Bus Selector : BusSelector  OutputSignals=Gyro_x_radDs,Gyro_y_radDs,Gyro_z_radDs
  Bus Selector1 : BusSelector  OutputSignals=Acc_x_mDs2,Acc_y_mDs2,Acc_z_mDs2
  Constant : Constant  Value=0  OutDataTypeStr=Bus: IMU_Bus
  IMU : Outport
  wires:
  Gyro_Raw/1 -> Bus Selector/1
  Acc_Raw/1 -> Bus Selector1/1
  Constant/1 -> Bus Assignment/1
  timestamp_ms/1 -> Bus Assignment/2
  Bus Assignment/1 -> IMU/1
  Bus Selector/1 -> Bus Assignment/3  "<Gyro_x_radDs>"
  Bus Selector/2 -> Bus Assignment/4  "<Gyro_y_radDs>"
  Bus Selector/3 -> Bus Assignment/5  "<Gyro_z_radDs>"
  Bus Selector1/1 -> Bus Assignment/6  "<Acc_x_mDs2>"
  Bus Selector1/2 -> Bus Assignment/7  "<Acc_y_mDs2>"
  Bus Selector1/3 -> Bus Assignment/8  "<Acc_z_mDs2>"

== system Plant/Sensor_Model/Sensor_IMU/Gyroscope ==
  States : Inport
  Errors_Enable : Inport  Port=2
  Vibration_Enable : Inport  Port=3
  Bus Assignment : Subsystem
  Physical_Model : Subsystem
  Sensor_Model : Subsystem
  Gyro_Raw : Outport
  wires:
  States/1 -> Physical_Model/1(States)
  Sensor_Model/1(y) -> Bus Assignment/1(Output)
  Bus Assignment/1(Gyro_Raw) -> Gyro_Raw/1
  Errors_Enable/1 -> Sensor_Model/1(Errors_Enable)
  Physical_Model/1(gyr_B_radDs) -> Sensor_Model/2(u)
  Vibration_Enable/1 -> Physical_Model/2(Vibration_Enable)

== system Plant/Sensor_Model/Sensor_MAG/Bus_Assignment ==
  Mag_Raw : Inport
  timestamp_ms : Inport  Port=2
  Bus Assignment : BusAssignment  AssignedSignals=timestamp,mag_x,mag_y,mag_z
  Bus Selector : BusSelector  OutputSignals=Mag_x_gauss,Mag_y_gauss,Mag_z_gauss
  Constant : Constant  Value=0  OutDataTypeStr=Bus: MAG_Bus
  Rate Transition : RateTransition  OutPortSampleTime=0.01
  MAG : Outport
  wires:
  Bus Assignment/1 -> Rate Transition/1
  Constant/1 -> Bus Assignment/1
  timestamp_ms/1 -> Bus Assignment/2
  Rate Transition/1 -> MAG/1
  Bus Selector/1 -> Bus Assignment/3  "<Mag_x_gauss>"
  Mag_Raw/1 -> Bus Selector/1
  Bus Selector/2 -> Bus Assignment/4  "<Mag_y_gauss>"
  Bus Selector/3 -> Bus Assignment/5  "<Mag_z_gauss>"

== system Plant/Sensor_Model/Sensor_MAG/Sensor_Magnetometer ==
  States : Inport
  Errors_Enable : Inport  Port=2
  Bus Assignment : Subsystem
  Physical_Model : Subsystem
  Sensor_Model : Subsystem
  Mag_Raw : Outport
  wires:
  Bus Assignment/1(Mag_Raw) -> Mag_Raw/1
  Sensor_Model/1(y) -> Bus Assignment/1(Output)
  States/1 -> Physical_Model/1(States)
  Physical_Model/1(mag_B_Gauss) -> Sensor_Model/2(u)
  Errors_Enable/1 -> Sensor_Model/1(Errors_Enable)

== system Plant/Actuators/Motors/ESCs/Calculate_Rotor_Speed ==
  u0 : Inport
  Add : Sum
  Compare To Constant : simulink/Logic and Bit Operations/Compare To Constant  relop=>  const=0.1  OutDataTypeStr=boolean
  Constant1 : Constant  Value=p  OutDataTypeStr=single
  Gain1 : Gain  Gain=k  OutDataTypeStr=Inherit: Same as input
  Multiply : Product
  Saturation1 : Saturate  UpperLimit=9999999  LowerLimit=0
  omega_B_radPs : Outport
  wires:
  Multiply/1 -> Saturation1/1
  Gain1/1 -> Add/1
  Saturation1/1 -> omega_B_radPs/1
  u0/1 -> Compare To Constant/1, Gain1/1
  Constant1/1 -> Add/2
  Compare To Constant/1 -> Multiply/1
  Add/1 -> Multiply/2

== system Plant/Actuators/Motors/ESCs/Signal_Unified ==
  Control_Out : Inport
  Constant : Constant  Value=1000  OutDataTypeStr=uint16
  Gain : Gain  Gain=0.001  OutDataTypeStr=single
  Saturation : Saturate  UpperLimit=2000  LowerLimit=1000
  Subtract : Sum  Inputs=+-  OutDataTypeStr=Inherit: Same as accumulator
  u0 : Outport
  wires:
  Constant/1 -> Subtract/2
  Control_Out/1 -> Saturation/1
  Saturation/1 -> Subtract/1
  Subtract/1 -> Gain/1
  Gain/1 -> u0/1

== system Plant/Actuators/Motors/Force/Thrust ==
  rotor_speed_radDs : Inport
  Multiply : Product  OutDataTypeStr=Inherit: Same as first input
  Square : Math  Operator=square  SaturateOnIntegerOverflow=on
  cT : Constant  Value=cT
  thrust_B_N : Outport
  wires:
  rotor_speed_radDs/1 -> Square/1
  Square/1 -> Multiply/1
  cT/1 -> Multiply/2
  Multiply/1 -> thrust_B_N/1

== system Plant/Actuators/Motors/Torque/Gyroscopic_Torque ==
  rotor_speed_radDs : Inport
  omega_B_radDs : Inport  Port=2
  Add : Sum  Inputs=--++
  Constant : Constant  Value=[0;0;Im]  OutDataTypeStr=single
  Demux : Demux
  Multiply : Product
  cross_product : AP_Math/cross_product  SystemSampleTime=-1
  gyroscopic_torque : Outport
  wires:
  Demux/1 -> Add/1
  Constant/1 -> cross_product/1
  Demux/4 -> Add/4
  Add/1 -> Multiply/1
  Demux/3 -> Add/3
  Demux/2 -> Add/2
  omega_B_radDs/1 -> Multiply/2
  Multiply/1 -> cross_product/2
  cross_product/1 -> gyroscopic_torque/1
  rotor_speed_radDs/1 -> Demux/1

== system Plant/Actuators/Motors/Torque/Rotor_Generated_Torque ==
  rotor_speed_radDs : Inport
  Multiply : Product  Multiplication=Matrix(*)
  Square : Math  Operator=square  SaturateOnIntegerOverflow=on
  X_Frame : Constant  Value=[-L*cT,L*cT,L*cT,-L*cT;L*cT,-L*cT,L*cT,-L*cT;cQ,cQ,-cQ,-cQ]  OutDataTypeStr=single
  rotor_torque : Outport
  wires:
  X_Frame/1 -> Multiply/1
  Square/1 -> Multiply/2
  Multiply/1 -> rotor_torque/1
  rotor_speed_radDs/1 -> Square/1

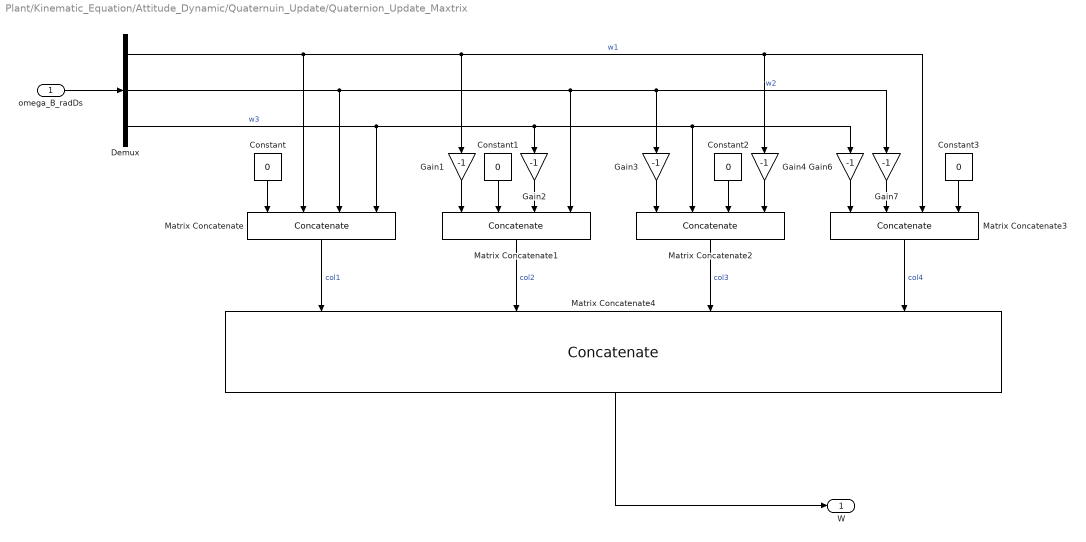
== system Plant/Kinematic_Equation/Attitude_Dynamic/Quaternuin_Update/Quaternion_Update_Maxtrix ==
  omega_B_radDs : Inport
  Constant{,1..3} (4 alike) : Constant  Value=0  OutDataTypeStr=single
  Demux : Demux  Outputs=3
  Gain{1..4,6..7} (6 alike) : Gain  Gain=-1  OutDataTypeStr=Inherit: Same as input
  Matrix Concatenate{,1..3} (4 alike) : Concatenate  NumInputs=4
  Matrix Concatenate4 : Concatenate  NumInputs=4  Mode=Multidimensional array  ConcatenateDimension=2
  W : Outport
  wires:
  Gain1/1 -> Matrix Concatenate1/1
  Gain7/1 -> Matrix Concatenate3/2
  Matrix Concatenate2/1 -> Matrix Concatenate4/3  "col3"
  Constant2/1 -> Matrix Concatenate2/3
  Matrix Concatenate4/1 -> W/1
  Demux/1 -> Gain1/1, Gain4/1, Matrix Concatenate3/3, Matrix Concatenate/2  "w1"
  Matrix Concatenate/1 -> Matrix Concatenate4/1  "col1"
  Matrix Concatenate1/1 -> Matrix Concatenate4/2  "col2"
  Constant3/1 -> Matrix Concatenate3/4
  Gain6/1 -> Matrix Concatenate3/1
  Constant1/1 -> Matrix Concatenate1/2
  Matrix Concatenate3/1 -> Matrix Concatenate4/4  "col4"
  Demux/2 -> Gain3/1, Gain7/1, Matrix Concatenate1/4, Matrix Concatenate/3  "w2"
  Constant/1 -> Matrix Concatenate/1
  Gain3/1 -> Matrix Concatenate2/1
  Demux/3 -> Gain2/1, Gain6/1, Matrix Concatenate2/2, Matrix Concatenate/4  "w3"
  Gain2/1 -> Matrix Concatenate1/3
  omega_B_radDs/1 -> Demux/1
  Gain4/1 -> Matrix Concatenate2/4

== system Plant/Sensor_Model/Sensor_Barometer/Sensor_Model/Routing ==
  Errors_Enable : Inport
  output_clean : Inport  Port=2
  output_error : Inport  Port=3
  Switch : Switch  Criteria=u2 > Threshold
  y : Outport
  wires:
  Switch/1 -> y/1
  output_error/1 -> Switch/1
  output_clean/1 -> Switch/3
  Errors_Enable/1 -> Switch/2

== system Plant/Sensor_Model/Sensor_Barometer/Sensor_Model/Sensor_Error ==
  u : Inport
  Constant3 : Constant  Value=Sensor_Model.Baro.Bias  VectorParams1D=off  OutDataTypeStr=single
  Sum : Sum  Inputs=|++  InputSameDT=on  OutDataTypeStr=Inherit: Same as first input
  y : Outport
  wires:
  Sum/1 -> y/1
  u/1 -> Sum/1
  Constant3/1 -> Sum/2

== system Plant/Sensor_Model/Sensor_GPS/Bus_Assignment/WGS84_Position ==
  pos_WGS84 : Inport
  Demux1 : Demux  Outputs=3
  Signal Conversion : SignalConversion  OverrideOpt=off
  Signal Conversion1 : SignalConversion  OverrideOpt=off
  Signal Conversion2 : SignalConversion  OverrideOpt=off
  lon : Outport
  lat : Outport  Port=2
  height : Outport  Port=3
  wires:
  Demux1/3 -> Signal Conversion2/1  "POS_h_WGS84"
  Signal Conversion/1 -> lon/1
  Demux1/1 -> Signal Conversion/1  "POS_lambda_WGS84"
  pos_WGS84/1 -> Demux1/1
  Demux1/2 -> Signal Conversion1/1  "POS_mue_WGS84"
  Signal Conversion1/1 -> lat/1
  Signal Conversion2/1 -> height/1

== system Plant/Sensor_Model/Sensor_GPS/Bus_Assignment/gSpeed_mDs ==
  u_O_mDs : Inport
  v_O_mDs : Inport  Port=2
  Add : Sum
  Math Function : Math  Operator=square  SaturateOnIntegerOverflow=on
  Math Function1 : Math  Operator=square  SaturateOnIntegerOverflow=on
  Saturation : Saturate  UpperLimit=inf  LowerLimit=0
  Sqrt : Sqrt  SaturateOnIntegerOverflow=on
  gSpeed_mPs : Outport
  wires:
  Sqrt/1 -> gSpeed_mPs/1
  Math Function/1 -> Add/1
  Math Function1/1 -> Add/2
  Saturation/1 -> Sqrt/1
  Add/1 -> Saturation/1
  u_O_mDs/1 -> Math Function/1
  v_O_mDs/1 -> Math Function1/1

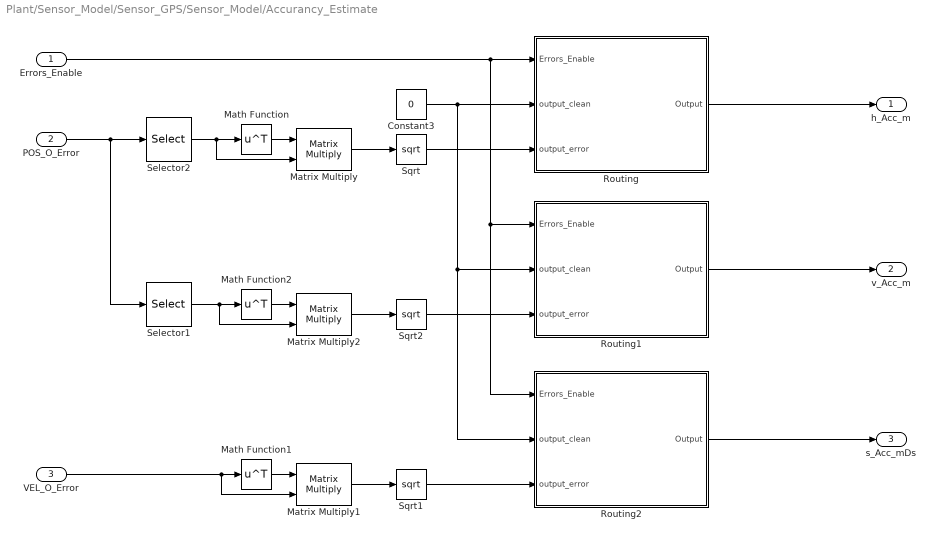
== system Plant/Sensor_Model/Sensor_GPS/Sensor_Model/Accurancy_Estimate ==
  Errors_Enable : Inport
  POS_O_Error : Inport  Port=2
  VEL_O_Error : Inport  Port=3
  Constant3 : Constant  Value=0
  Math Function : Math  Operator=transpose  SaturateOnIntegerOverflow=on
  Math Function1 : Math  Operator=transpose  SaturateOnIntegerOverflow=on
  Math Function2 : Math  Operator=transpose  SaturateOnIntegerOverflow=on
  Matrix Multiply : Product  Multiplication=Matrix(*)
  Matrix Multiply1 : Product  Multiplication=Matrix(*)
  Matrix Multiply2 : Product  Multiplication=Matrix(*)
  Routing : Subsystem
  Routing1 : Subsystem
  Routing2 : Subsystem
  Selector1 : Selector  InputPortWidth=3  IndexOptions=Index vector (dialog)  Indices=3  OutputSizes=1
  Selector2 : Selector  InputPortWidth=3  IndexOptions=Index vector (dialog)  Indices=[1 2]  OutputSizes=1
  Sqrt : Sqrt  OutputSignalType=real  SaturateOnIntegerOverflow=on
  Sqrt1 : Sqrt  OutputSignalType=real  SaturateOnIntegerOverflow=on
  Sqrt2 : Sqrt  OutputSignalType=real  SaturateOnIntegerOverflow=on
  h_Acc_m : Outport
  v_Acc_m : Outport  Port=2
  s_Acc_mDs : Outport  Port=3
  wires:
  Sqrt1/1 -> Routing2/3(output_error)
  Routing/1(Output) -> h_Acc_m/1
  Errors_Enable/1 -> Routing2/1(Errors_Enable), Routing1/1(Errors_Enable), Routing/1(Errors_Enable)
  POS_O_Error/1 -> Selector1/1, Selector2/1
  Sqrt/1 -> Routing/3(output_error)
  Constant3/1 -> Routing2/2(output_clean), Routing1/2(output_clean), Routing/2(output_clean)
  Routing1/1(Output) -> v_Acc_m/1
  Selector1/1 -> Math Function2/1, Matrix Multiply2/2
  Routing2/1(Output) -> s_Acc_mDs/1
  Math Function1/1 -> Matrix Multiply1/1
  Math Function2/1 -> Matrix Multiply2/1
  Math Function/1 -> Matrix Multiply/1
  Selector2/1 -> Matrix Multiply/2, Math Function/1
  Matrix Multiply1/1 -> Sqrt1/1
  Sqrt2/1 -> Routing1/3(output_error)
  Matrix Multiply/1 -> Sqrt/1
  Matrix Multiply2/1 -> Sqrt2/1
  VEL_O_Error/1 -> Matrix Multiply1/2, Math Function1/1
